simulink model "telemed_screening"  (R2026a)
settings: Solver=ode45  StopTime=2000
settings Model: Creator=Abhishekh  LastModifiedBy=Abhishekh

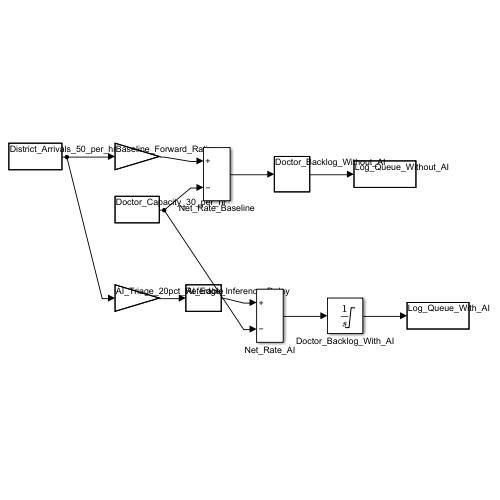
[thumbnail: Simulink's stored preview of the top-level diagram]
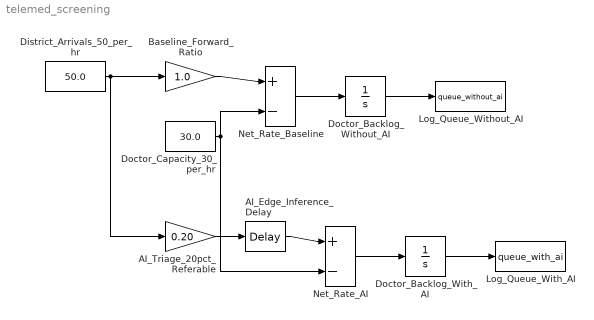
== system telemed_screening ==
  AI_Edge_Inference_Delay : TransportDelay  DelayTime=0.00014
  AI_Triage_20pct_Referable : Gain  Gain=0.20
  Baseline_Forward_Ratio : Gain  Gain=1.0
  District_Arrivals_50_per_hr : Constant  Value=50.0
  Doctor_Backlog_With_AI : Integrator  LimitOutput=on  LowerSaturationLimit=0
  Doctor_Backlog_Without_AI : Integrator  LimitOutput=on  LowerSaturationLimit=0
  Doctor_Capacity_30_per_hr : Constant  Value=30.0
  Log_Queue_With_AI : ToWorkspace  VariableName=queue_with_ai  SampleTime=-1
  Log_Queue_Without_AI : ToWorkspace  VariableName=queue_without_ai  SampleTime=-1
  Net_Rate_AI : Sum  Inputs=+-
  Net_Rate_Baseline : Sum  Inputs=+-
  wires:
  District_Arrivals_50_per_hr/1 -> Baseline_Forward_Ratio/1, AI_Triage_20pct_Referable/1
  Baseline_Forward_Ratio/1 -> Net_Rate_Baseline/1
  Doctor_Capacity_30_per_hr/1 -> Net_Rate_Baseline/2, Net_Rate_AI/2
  Net_Rate_Baseline/1 -> Doctor_Backlog_Without_AI/1
  Doctor_Backlog_Without_AI/1 -> Log_Queue_Without_AI/1
  AI_Triage_20pct_Referable/1 -> AI_Edge_Inference_Delay/1
  AI_Edge_Inference_Delay/1 -> Net_Rate_AI/1
  Net_Rate_AI/1 -> Doctor_Backlog_With_AI/1
  Doctor_Backlog_With_AI/1 -> Log_Queue_With_AI/1
